simulink model "sim_quadrotor"  (R2015a)
settings: Solver=ode3  StartTime=0  StopTime=inf  FixedStep=sampleTime_qcsim  MaxStep=0.1  RelTol=1e-3
InitFcn:
  | % load parameters of the default quadrotor
  | disp('Quadrotor parameters loaded by InitFcn')
  | paramsFilters %load mdl_quadcopter as well!
  | 
  | % change to Simulation folder if in data folder
  | cd([matlabpath '/Simulation']);
undefined symbols (not defined in the file): altEstim, controlParams, Discrete, ofhandle, quad, quadEDT, sampleTime_qcsim, Time, vishandle
libraries: simulink x25, ctrlSharedLib x3, commnoisgen2 x1
settings Model: CovSFcnEnable=off  Creator=corkep  LastModifiedBy=student
settings DataIOCC: LimitDataPoints=off  SaveFormat=StructureWithTime  SignalLoggingSaveFormat=ModelDataLogs  SignalLogging=off  DSMLogging=off
settings OptimizationCC: ExpressionDepthLimit=2147483647  OptimizeModelRefInitCode=on  LifeSpan=1
settings DebuggingCC: UnderspecifiedInitializationDetection=Classic  MergeDetectMultiDrivingBlocksExec=none  SolverPrmCheckMsg=warning  FcnCallInpInsideContextMsg=UseLocalSettings  StateNameClashWarn=warning
settings HardwareCC: TargetBitPerLong=64  TargetBitPerPointer=64  TargetLongLongMode=on  TargetIntDivRoundTo=Zero  TargetEndianess=LittleEndian  TargetWordSize=64  TargetHWDeviceType=MATLAB Host  ProdEqTarget=off
settings RTWCC: SystemTargetFile=ert_shrlib.tlc  GenCodeOnly=on  MakeCommand="make_rtw OPTS=\"-DDEFAULT_BUFFER_SIZE=4600\""  GenerateMakefile=off  TemplateMakefile=ert_default_tmf  Description=Embedded Coder (host-based shared library target)  BuildConfiguration=Faster Runs  RTWCompilerOptimization=on
settings CodeAppCC: IgnoreCustomStorageClasses=off
settings STFCustomTargetCC: ParMdlRefBuildCompliant=on  CompOptLevelCompliant=on  IncludeMdlTerminateFcn=off  CombineOutputUpdateFcns=on  MatFileLogging=on  MultiInstanceERTCode=on  CodeInterfacePackaging=Reusable function  SupportContinuousTime=off  SupportVariableSizeSignals=off  ModelStepFunctionPrototypeControlCompliant=on  SystemTargetFile=ert_shrlib.tlc
settings ERTTargetCC: ParMdlRefBuildCompliant=on  CompOptLevelCompliant=on  IncludeMdlTerminateFcn=off  MatFileLogging=on  MultiInstanceERTCode=on  CodeInterfacePackaging=Reusable function  SupportContinuousTime=off  SupportVariableSizeSignals=off  ModelStepFunctionPrototypeControlCompliant=on  MultiInstanceErrorCode=Warning  ERTCustomFileTemplate=example_file_process.tlc

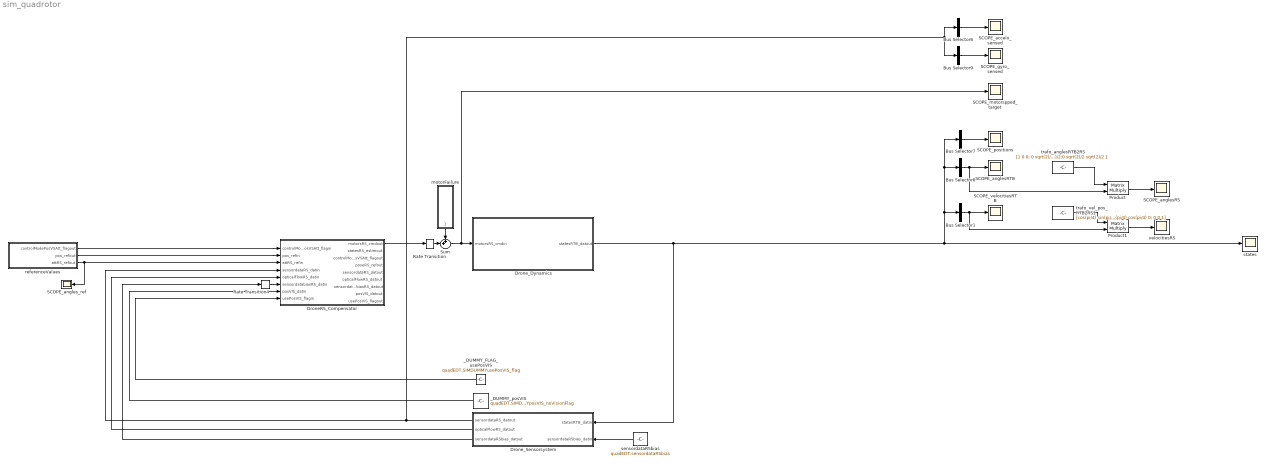
== system sim_quadrotor ==
  Bus Selector1 : BusSelector  OutputSignals=dx,dy,dz  OutputAsBus=on
  Bus Selector6 : BusSelector  OutputSignals=ddx,ddy,ddz  OutputAsBus=on
  Bus Selector7 : BusSelector  OutputSignals=X,Y,Z  OutputAsBus=on
  Bus Selector8 : BusSelector  OutputSignals=yaw,pitch,roll  OutputAsBus=on
  Bus Selector9 : BusSelector  OutputSignals=p,q,r  OutputAsBus=on
  DroneRS_Compensator : Subsystem  TreatAsAtomicUnit=on
  Drone_Dynamics : Subsystem  AncestorBlock=roblocks/Dynamics/Quadrotor
  Drone_Sensorsystem : Subsystem
  Product : Product  Multiplication=Matrix(*)
  Product1 : Product  Multiplication=Matrix(*)
  Rate Transition : RateTransition
  Rate Transition4 : RateTransition  OutPortSampleTime=sampleTime_qcsim
  SCOPE_accelo_sensed : Scope
      settings: TimeRange=14.995  YMin=-13  YMax=2  SaveName=ScopeData11
  SCOPE_anglesRS : Scope
      settings: TimeRange=9.635  YMin=-0.2  YMax=0.1  SaveName=ScopeData8
  SCOPE_anglesRTB : Scope
      settings: TimeRange=10.425  YMin=-0.04  YMax=0.11  SaveName=ScopeData5
  SCOPE_angles_ref : Scope
      settings: TimeRange=15  YMin=-0.15  YMax=0.2  SaveName=ScopeData28
  SCOPE_gyro_sensed : Scope
      settings: TimeRange=14.995  YMin=-0.002  YMax=0.00175  SaveName=ScopeData10
  SCOPE_motorspped_target : Scope
      settings: TimeRange=9.040000000000001  YMin=-400  YMax=400  SaveName=ScopeData2
  SCOPE_positions : Scope
      settings: TimeRange=9.040000000000001  YMin=-1.5  YMax=0.5  SaveName=ScopeData3
  SCOPE_velocitiesRTB : Scope
      settings: TimeRange=13.045  YMin=-1.5  YMax=0.5  SaveName=ScopeData22
  Sum : Sum  Inputs=++|
  _DUMMY_FLAG_usePosVIS : Constant  Value=quadEDT.SIMDUMMYusePosVIS_flag
  _DUMMY_posVIS : Constant  Value=quadEDT.SIMDUMMYposVIS_noVisionFlag
  motorFailure : Subsystem
  referenceValues : Subsystem
  sensordataRSbias : Constant  Value=quadEDT.sensordataRSbias
  states : Scope
      settings: TimeRange=20  YMin=-0.005  YMax=0.055  SaveName=ScopeData7
  trafo_anglesRTB2RS : Constant  Value=[1 0 0; 0 sqrt(2)/2 -sqrt(2)/2;0 sqrt(2)/2 sqrt(2)/2 ]
  trafo_vel_pos_RTB2RS1 : Constant  Value=[cos(pi/4) sin(pi/4) 0 ; -sin(pi/4) cos(pi/4) 0; 0 0 1]
  velocitiesRS : Scope
      settings: TimeRange=8.18  YMin=-4.991831340204151  YMax=1.573556915322435  SaveName=ScopeData39
  wires:
  Bus Selector7/1 -> SCOPE_positions/1
  Bus Selector8/1 -> Product/2, SCOPE_anglesRTB/1
  Bus Selector6/1 -> SCOPE_accelo_sensed/1
  Bus Selector9/1 -> SCOPE_gyro_sensed/1
  DroneRS_Compensator/1(motorsRS_cmdout) -> Rate Transition/1
  referenceValues/2("pos_refout ") -> DroneRS_Compensator/2(pos_refin)
  Sum/1 -> SCOPE_motorspped_target/1, Drone_Dynamics/1(motorsRS_cmdin)
  motorFailure/1(motorRS_cmdout) -> Sum/1
  Rate Transition/1 -> Sum/2
  referenceValues/1(controlModePosVSAtt_flagout) -> DroneRS_Compensator/1(controlModePosVSAtt_flagin)
  referenceValues/3(attRS_refout) -> DroneRS_Compensator/3(attRS_refin), SCOPE_angles_ref/1
  Drone_Dynamics/1(statesRTB_datout) -> Drone_Sensorsystem/1(statesRTB_datin), states/1, Bus Selector1/1, Bus Selector8/1, Bus Selector7/1
  sensordataRSbias/1 -> Drone_Sensorsystem/2(sensordataRSbias_datin)
  Drone_Sensorsystem/2(opticalFlowRS_datout) -> DroneRS_Compensator/5(opticalFlowRS_datin)
  Rate Transition4/1 -> DroneRS_Compensator/6(sensordatabiasRS_datin)
  Drone_Sensorsystem/1(sensordataRS_datout) -> DroneRS_Compensator/4(sensordataRS_datin), Bus Selector9/1, Bus Selector6/1
  Drone_Sensorsystem/3(sensordataRSbias_datout) -> Rate Transition4/1
  Product/1 -> SCOPE_anglesRS/1
  trafo_anglesRTB2RS/1 -> Product/1
  _DUMMY_posVIS/1 -> DroneRS_Compensator/7(posVIS_datin)
  Bus Selector1/1 -> Product1/2, SCOPE_velocitiesRTB/1
  Product1/1 -> velocitiesRS/1
  _DUMMY_FLAG_usePosVIS/1 -> DroneRS_Compensator/8(usePosVIS_flagin)
  trafo_vel_pos_RTB2RS1/1 -> Product1/1

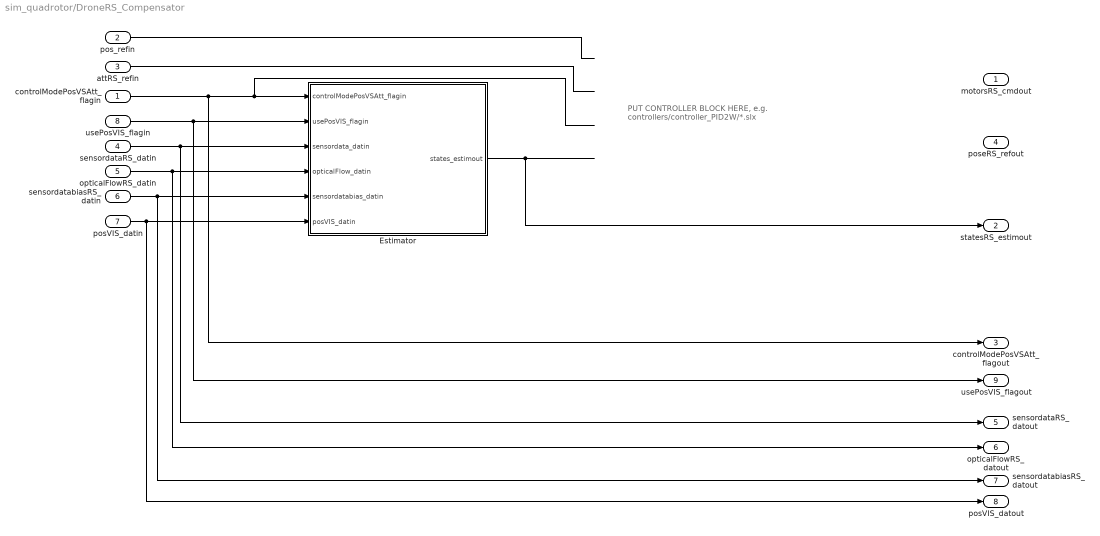
== system sim_quadrotor/DroneRS_Compensator ==
  note: PUT CONTROLLER BLOCK HERE,
      | e.g. controllers/controller_PID2W/*.slx
  controlModePosVSAtt_flagin : Inport
  pos_refin : Inport  Port=2
  attRS_refin : Inport  Port=3
  sensordataRS_datin : Inport  Port=4
  opticalFlowRS_datin : Inport  Port=5
  sensordatabiasRS_datin : Inport  Port=6
  posVIS_datin : Inport  Port=7
  usePosVIS_flagin : Inport  Port=8
  Estimator : Subsystem
  motorsRS_cmdout : Outport
  statesRS_estimout : Outport  Port=2
  controlModePosVSAtt_flagout : Outport  Port=3
  poseRS_refout : Outport  Port=4
  sensordataRS_datout : Outport  Port=5
  opticalFlowRS_datout : Outport  Port=6
  sensordatabiasRS_datout : Outport  Port=7
  posVIS_datout : Outport  Port=8
  usePosVIS_flagout : Outport  Port=9
  wires:
  sensordataRS_datin/1 -> sensordataRS_datout/1, Estimator/3(sensordata_datin)
  pos_refin/1 -> ?
  Estimator/1(states_estimout) -> statesRS_estimout/1
  attRS_refin/1 -> ?
  controlModePosVSAtt_flagin/1 -> controlModePosVSAtt_flagout/1, Estimator/1(controlModePosVSAtt_flagin)
  sensordatabiasRS_datin/1 -> Estimator/5(sensordatabias_datin), sensordatabiasRS_datout/1
  opticalFlowRS_datin/1 -> Estimator/4(opticalFlow_datin), opticalFlowRS_datout/1
  posVIS_datin/1 -> Estimator/6(posVIS_datin), posVIS_datout/1
  ? -> motorsRS_cmdout/1
  usePosVIS_flagin/1 -> usePosVIS_flagout/1, Estimator/2(usePosVIS_flagin)
  ? -> poseRS_refout/1

== system sim_quadrotor/Drone_Dynamics ==
  motorsRS_cmdin : Inport
  Bus Creator : BusCreator  Inputs='X','Y','Z','yaw','pitch','roll','dx','dy','dz','p','q','r'
  Demux : Demux  Outputs=12
  Dynamics (Robotics Toolbox Peter Corke) : S-Function  FunctionName=quadrotor_dynamics  Parameters=quad
  MotorsRSToW : Subsystem
  statesRTB_datout : Outport
  wires:
  Demux/1 -> Bus Creator/1  "X"
  Demux/3 -> Bus Creator/3  "Z"
  Demux/4 -> Bus Creator/4  "yaw"
  Demux/5 -> Bus Creator/5  "pitch"
  motorsRS_cmdin/1 -> MotorsRSToW/1(motorsRS_cmdin)
  Demux/7 -> Bus Creator/7  "dx"
  Demux/9 -> Bus Creator/9  "dz"
  Demux/2 -> Bus Creator/2  "Y"
  Demux/6 -> Bus Creator/6  "roll"
  Demux/8 -> Bus Creator/8  "dy"
  Bus Creator/1 -> statesRTB_datout/1
  Dynamics (Robotics Toolbox Peter Corke)/1 -> Demux/1
  Demux/10 -> Bus Creator/10  "p"
  Demux/11 -> Bus Creator/11  "q"
  Demux/12 -> Bus Creator/12  "r"
  MotorsRSToW/1(omega_cmdout) -> Dynamics (Robotics Toolbox Peter Corke)/1

== system sim_quadrotor/Drone_Sensorsystem ==
  statesRTB_datin : Inport
  sensordataRSbias_datin : Inport  Port=2
  IMU_Pressure : Subsystem
  Rate Transition1 : RateTransition  OutPortSampleTime=sampleTime_qcsim
  Rate Transition2 : RateTransition  OutPortSampleTime=sampleTime_qcsim
  camera : Subsystem
  sensordataRS_datout : Outport
  opticalFlowRS_datout : Outport  Port=2
  sensordataRSbias_datout : Outport  Port=3
  wires:
  statesRTB_datin/1 -> IMU_Pressure/2(statesRTB_datin), camera/1(statesRTB_datin)
  sensordataRSbias_datin/1 -> sensordataRSbias_datout/1, IMU_Pressure/1(sensordataRSbias_datin)
  Rate Transition2/1 -> sensordataRS_datout/1
  Rate Transition1/1 -> opticalFlowRS_datout/1
  IMU_Pressure/1(sensordataRS_datout) -> Rate Transition2/1
  camera/1(opticalFlowRS_datout) -> Rate Transition1/1

== system sim_quadrotor/motorFailure ==
  Constant : Constant  Value=0
  Constant1 : Constant  Value=0
  Mux1 : Mux
  Step : Step  Time=quadEDT.motorFailure_time  SampleTime=0
  Step1 : Step  Time=quadEDT.motorFailure_time + quadEDT.motorFailure_duration  SampleTime=0
  Sum : Sum  Inputs=|+-
  motorFailure_gainm2 : Gain  Gain=quadEDT.motorFailure_gainm2
  motorFailure_gainm3 : Gain  Gain=quadEDT.motorFailure_gainm3
  motorRS_cmdout : Outport
  wires:
  Step/1 -> Sum/1
  Step1/1 -> Sum/2
  Sum/1 -> motorFailure_gainm3/1, motorFailure_gainm2/1
  Constant/1 -> Mux1/1
  motorFailure_gainm2/1 -> Mux1/2
  motorFailure_gainm3/1 -> Mux1/3
  Constant1/1 -> Mux1/4
  Mux1/1 -> motorRS_cmdout/1

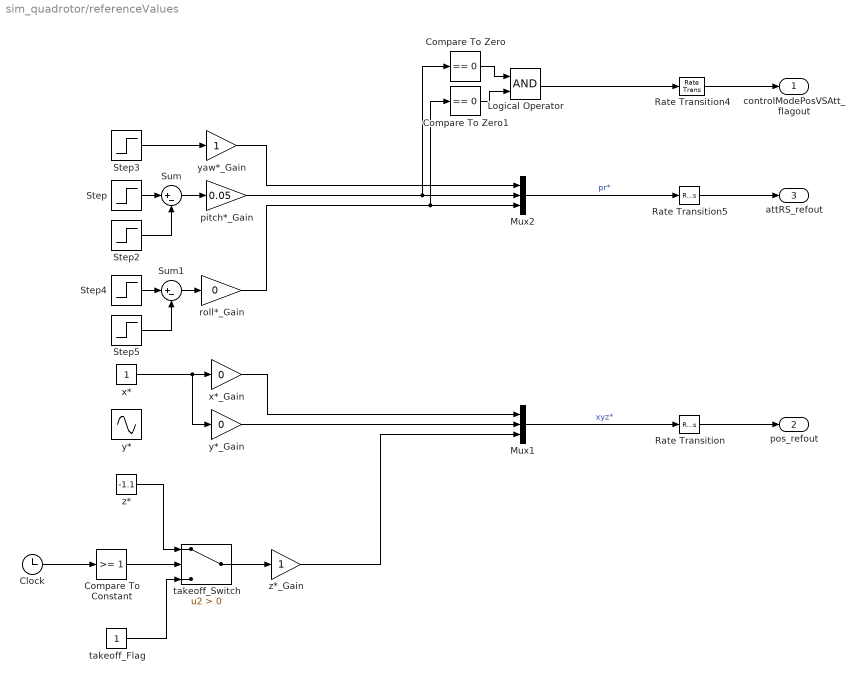
== system sim_quadrotor/referenceValues ==
  Clock : Clock
  Compare To Constant : simulink/Logic and Bit Operations/Compare To Constant  relop=>=  const=1  OutDataTypeStr=boolean
  Compare To Zero : simulink/Logic and Bit Operations/Compare To Zero  relop===  OutDataTypeStr=boolean
  Compare To Zero1 : simulink/Logic and Bit Operations/Compare To Zero  relop===  OutDataTypeStr=boolean
  Logical Operator : Logic  AllPortsSameDT=off  OutDataTypeStr=boolean
  Mux1 : Mux  Inputs=3
  Mux2 : Mux  Inputs=3
  Rate Transition : RateTransition  OutPortSampleTime=sampleTime_qcsim
  Rate Transition4 : RateTransition  OutPortSampleTime=sampleTime_qcsim
  Rate Transition5 : RateTransition  OutPortSampleTime=sampleTime_qcsim
  Step : Step  SampleTime=0
  Step2 : Step  Time=2  SampleTime=0
  Step3 : Step  Time=4.5  After=0.1  SampleTime=0
  Step4 : Step  SampleTime=0
  Step5 : Step  Time=2  SampleTime=0
  Sum : Sum  Inputs=|+-
  Sum1 : Sum  Inputs=|+-
  pitch*_Gain : Gain  Gain=0.05
  roll*_Gain : Gain  Gain=0
  takeoff_Flag : Constant  SampleTime=0
  takeoff_Switch : Switch  Criteria=u2 > Threshold
  x* : Constant  SampleTime=0
  x*_Gain : Gain  Gain=0
  y* : Sin  Frequency=2*pi*.125  SampleTime=0
  y*_Gain : Gain  Gain=0
  yaw*_Gain : Gain
  z* : Constant  Value=-1.1  SampleTime=0
  z*_Gain : Gain
  controlModePosVSAtt_flagout : Outport
  "pos_refout " : Outport  Port=2
  attRS_refout : Outport  Port=3
  wires:
  z*/1 -> takeoff_Switch/1
  y*_Gain/1 -> Mux1/2
  x*/1 -> y*_Gain/1, x*_Gain/1
  Mux1/1 -> Rate Transition/1  "xyz*"
  x*_Gain/1 -> Mux1/1
  Rate Transition/1 -> "pos_refout "/1
  Rate Transition4/1 -> controlModePosVSAtt_flagout/1
  Step/1 -> Sum/1
  Mux2/1 -> Rate Transition5/1  "pr*"
  Sum1/1 -> roll*_Gain/1
  Rate Transition5/1 -> attRS_refout/1
  Sum/1 -> pitch*_Gain/1
  Step2/1 -> Sum/2
  yaw*_Gain/1 -> Mux2/1
  pitch*_Gain/1 -> Mux2/2, Compare To Zero/1
  roll*_Gain/1 -> Mux2/3, Compare To Zero1/1
  Compare To Zero/1 -> Logical Operator/1
  Compare To Zero1/1 -> Logical Operator/2
  Logical Operator/1 -> Rate Transition4/1
  Step3/1 -> yaw*_Gain/1
  Clock/1 -> Compare To Constant/1
  Compare To Constant/1 -> takeoff_Switch/2
  takeoff_Flag/1 -> takeoff_Switch/3
  takeoff_Switch/1 -> z*_Gain/1
  z*_Gain/1 -> Mux1/3
  Step4/1 -> Sum1/1
  Step5/1 -> Sum1/2

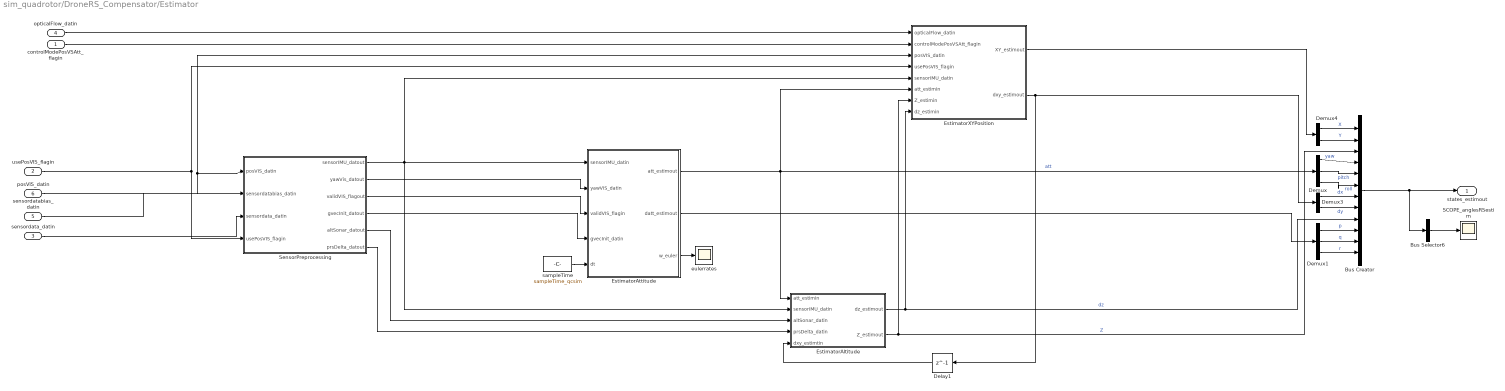
== system sim_quadrotor/DroneRS_Compensator/Estimator ==
  controlModePosVSAtt_flagin : Inport
  usePosVIS_flagin : Inport  Port=2
  sensordata_datin : Inport  Port=3
  opticalFlow_datin : Inport  Port=4
  sensordatabias_datin : Inport  Port=5
  posVIS_datin : Inport  Port=6
  Bus Creator : BusCreator  Inputs='X','Y','Z','yaw','pitch','roll','dx','dy','dz','p','q','r'
  Bus Selector6 : BusSelector  OutputSignals=yaw,pitch,roll  OutputAsBus=on
  Delay1 : Delay  DelayLength=1  InitialCondition=0
  Demux : Demux  Outputs=3
  Demux1 : Demux  Outputs=3
  Demux3 : Demux  Outputs=2
  Demux4 : Demux  Outputs=2
  EstimatorAltitude : Subsystem
  EstimatorAttitude : MATLAB Function  TreatAsAtomicUnit=on
  EstimatorXYPosition : Subsystem
  SCOPE_anglesRSestim : Scope
      settings: TimeRange=3.57  YMin=-0.08  YMax=0.06000000000000001  SaveName=ScopeData4
  SensorPreprocessing : Subsystem
  eulerrates : Scope
      settings: SaveName=ScopeData18
  sampleTime : Constant  Value=sampleTime_qcsim
  states_estimout : Outport
  wires:
  Bus Creator/1 -> Bus Selector6/1, states_estimout/1
  sampleTime/1 -> EstimatorAttitude/5(dt)
  sensordatabias_datin/1 -> SensorPreprocessing/2(sensordatabias_datin)
  EstimatorAttitude/3(w_euler) -> eulerrates/1
  EstimatorAltitude/2(Z_estimout) -> Bus Creator/3, EstimatorXYPosition/7(Z_estimin)  "Z"
  EstimatorAltitude/1(dz_estimout) -> Bus Creator/9, EstimatorXYPosition/8(dz_estimin)  "dz"
  opticalFlow_datin/1 -> EstimatorXYPosition/1(opticalFlow_datin)
  Demux3/1 -> Bus Creator/7  "dx"
  Demux3/2 -> Bus Creator/8  "dy"
  EstimatorXYPosition/2(dxy_estimout) -> Delay1/1, Demux3/1
  Delay1/1 -> EstimatorAltitude/5(dxy_estimtin)
  controlModePosVSAtt_flagin/1 -> EstimatorXYPosition/2(controlModePosVSAtt_flagin)
  Demux4/1 -> Bus Creator/1  "X"
  Demux4/2 -> Bus Creator/2  "Y"
  EstimatorXYPosition/1(XY_estimout) -> Demux4/1
  posVIS_datin/1 -> EstimatorXYPosition/3(posVIS_datin), SensorPreprocessing/1(posVIS_datin)
  usePosVIS_flagin/1 -> SensorPreprocessing/4(usePosVIS_flagin), EstimatorXYPosition/4(usePosVIS_flagin)
  Bus Selector6/1 -> SCOPE_anglesRSestim/1
  SensorPreprocessing/1(sensorIMU_datout) -> EstimatorAltitude/2(sensorIMU_datin), EstimatorXYPosition/5(sensorIMU_datin), EstimatorAttitude/1(sensorIMU_datin)
  SensorPreprocessing/4(gvecInit_datout) -> EstimatorAttitude/4(gvecInit_datin)
  sensordata_datin/1 -> SensorPreprocessing/3(sensordata_datin)
  SensorPreprocessing/5(altSonar_datout) -> EstimatorAltitude/3(altSonar_datin)
  SensorPreprocessing/6(prsDelta_datout) -> EstimatorAltitude/4(prsDelta_datin)
  EstimatorAttitude/1(att_estimout) -> EstimatorAltitude/1(att_estimin), Demux/1, EstimatorXYPosition/6(att_estimin)  "att"
  Demux/1 -> Bus Creator/4  "yaw"
  Demux/2 -> Bus Creator/5  "pitch"
  Demux/3 -> Bus Creator/6  "roll"
  Demux1/1 -> Bus Creator/10  "p"
  Demux1/2 -> Bus Creator/11  "q"
  Demux1/3 -> Bus Creator/12  "r"
  EstimatorAttitude/2(datt_estimout) -> Demux1/1
  SensorPreprocessing/3(validVIS_flagout) -> EstimatorAttitude/3(validVIS_flagin)
  SensorPreprocessing/2(yawVis_datout) -> EstimatorAttitude/2(yawVIS_datin)

== system sim_quadrotor/Drone_Dynamics/MotorsRSToW ==
  motorsRS_cmdin : Inport
  Signed Sqrt : Sqrt  Operator=signedSqrt  SaturateOnIntegerOverflow=on
  motorsRSToW2_Gain : Gain  Gain=quadEDT.motorsRSToW2_Gain
  omega_cmdout : Outport
  wires:
  motorsRSToW2_Gain/1 -> Signed Sqrt/1
  motorsRS_cmdin/1 -> motorsRSToW2_Gain/1
  Signed Sqrt/1 -> omega_cmdout/1

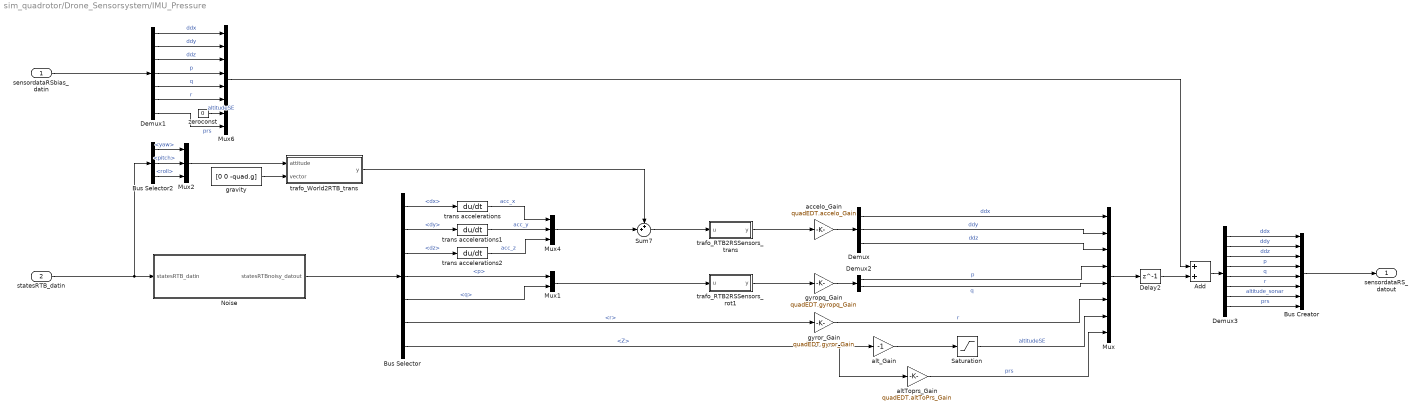
== system sim_quadrotor/Drone_Sensorsystem/IMU_Pressure ==
  sensordataRSbias_datin : Inport
  statesRTB_datin : Inport  Port=2
  " Noise" : Subsystem
  Add : Sum
  Bus Creator : BusCreator  Inputs=8
  Bus Selector : BusSelector  OutputSignals=dx,dy,dz,p,q,r,Z
  Bus Selector2 : BusSelector  OutputSignals=yaw,pitch,roll
  Delay2 : Delay  DelayLength=1  InitialCondition=0
  Demux : Demux  Outputs=3
  Demux1 : Demux  Outputs=7
  Demux2 : Demux  Outputs=2
  Demux3 : Demux  Outputs=8
  Mux : Mux  Inputs=8
  Mux1 : Mux  Inputs=2
  Mux2 : Mux  Inputs=3
  Mux4 : Mux  Inputs=3
  Mux6 : Mux  Inputs=8
  Saturation : Saturate  UpperLimit=inf  LowerLimit=quadEDT.altSenor_LowerLimit
  Sum7 : Sum  Inputs=++|
  accelo_Gain : Gain  Gain=quadEDT.accelo_Gain
  altToprs_Gain : Gain  Gain=quadEDT.altToPrs_Gain
  alt_Gain : Gain  Gain=-1
  gravity : Constant  Value=[0 0 -quad.g]
  gyropq_Gain : Gain  Gain=quadEDT.gyropq_Gain
  gyror_Gain : Gain  Gain=quadEDT.gyror_Gain
  trafo_RTB2RSSensors_rot1 : MATLAB Function  TreatAsAtomicUnit=on
  trafo_RTB2RSSensors_trans : MATLAB Function  TreatAsAtomicUnit=on
  trafo_World2RTB_trans : MATLAB Function  TreatAsAtomicUnit=on
  trans accelerations : Derivative
  trans accelerations1 : Derivative
  trans accelerations2 : Derivative
  zeroconst : Constant  Value=0
  sensordataRS_datout : Outport
  wires:
  statesRTB_datin/1 -> " Noise"/1(statesRTB_datin), Bus Selector2/1
  sensordataRSbias_datin/1 -> Demux1/1
  Demux2/2 -> Mux/5  "q"
  Demux2/1 -> Mux/4  "p"
  " Noise"/1(statesRTBnoisy_datout) -> Bus Selector/1
  Bus Selector/2 -> trans accelerations1/1  "<dy>"
  trans accelerations2/1 -> Mux4/3  "acc_z"
  trafo_RTB2RSSensors_trans/1(y) -> accelo_Gain/1
  Demux/1 -> Mux/1  "ddx"
  Demux/2 -> Mux/2  "ddy"
  gyror_Gain/1 -> Mux/6  "r"
  trans accelerations/1 -> Mux4/1  "acc_x"
  trans accelerations1/1 -> Mux4/2  "acc_y"
  Bus Selector2/1 -> Mux2/1  "<yaw>"
  Bus Selector2/2 -> Mux2/2  "<pitch>"
  Bus Selector2/3 -> Mux2/3  "<roll>"
  Demux/3 -> Mux/3  "ddz"
  Mux2/1 -> trafo_World2RTB_trans/1(attitude)
  gravity/1 -> trafo_World2RTB_trans/2(vector)
  trafo_World2RTB_trans/1(y) -> Sum7/1
  Sum7/1 -> trafo_RTB2RSSensors_trans/1(u)
  Mux4/1 -> Sum7/2
  Mux1/1 -> trafo_RTB2RSSensors_rot1/1(u)
  Bus Selector/4 -> Mux1/1  "<p>"
  Bus Selector/5 -> Mux1/2  "<q>"
  Bus Selector/6 -> gyror_Gain/1  "<r>"
  Bus Selector/7 -> altToprs_Gain/1, alt_Gain/1  "<Z>"
  alt_Gain/1 -> Saturation/1
  Saturation/1 -> Mux/7  "altitudeSE"
  Bus Selector/3 -> trans accelerations2/1  "<dz>"
  altToprs_Gain/1 -> Mux/8  "prs"
  Demux1/1 -> Mux6/1  "ddx"
  Demux1/2 -> Mux6/2  "ddy"
  Demux1/3 -> Mux6/3  "ddz"
  Demux1/4 -> Mux6/4  "p"
  Demux1/5 -> Mux6/5  "q"
  Demux1/6 -> Mux6/6  "r"
  zeroconst/1 -> Mux6/7  "altitudeSE"
  Demux1/7 -> Mux6/8  "prs"
  Mux6/1 -> Add/1
  Add/1 -> Demux3/1
  Mux/1 -> Delay2/1
  Demux3/3 -> Bus Creator/3  "ddz"
  Demux3/1 -> Bus Creator/1  "ddx"
  Demux3/2 -> Bus Creator/2  "ddy"
  Demux3/4 -> Bus Creator/4  "p"
  Demux3/5 -> Bus Creator/5  "q"
  Demux3/6 -> Bus Creator/6  "r"
  Demux3/7 -> Bus Creator/7  "altitude_sonar"
  Demux3/8 -> Bus Creator/8  "prs"
  Bus Creator/1 -> sensordataRS_datout/1
  trafo_RTB2RSSensors_rot1/1(y) -> gyropq_Gain/1
  Bus Selector/1 -> trans accelerations/1  "<dx>"
  Delay2/1 -> Add/2
  accelo_Gain/1 -> Demux/1
  gyropq_Gain/1 -> Demux2/1

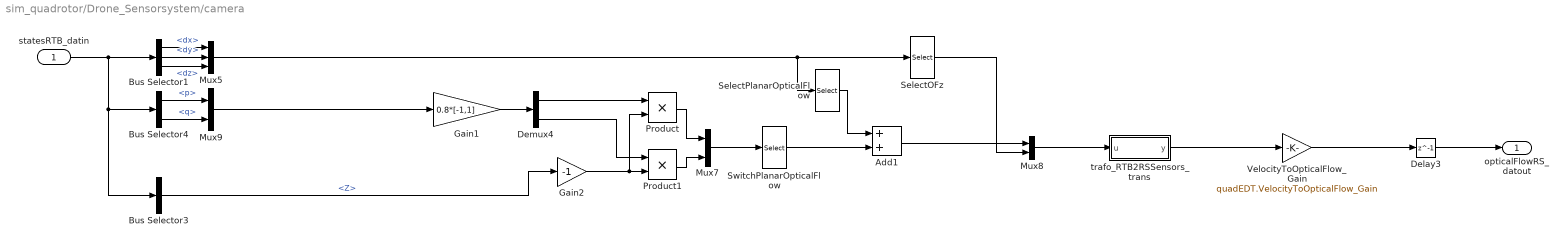
== system sim_quadrotor/Drone_Sensorsystem/camera ==
  statesRTB_datin : Inport
  Add1 : Sum
  Bus Selector1 : BusSelector  OutputSignals=dx,dy,dz
  Bus Selector3 : BusSelector  OutputSignals=Z
  Bus Selector4 : BusSelector  OutputSignals=p,q
  Delay3 : Delay  DelayLength=1  InitialCondition=0
  Demux4 : Demux  Outputs=2
  Gain1 : Gain  Gain=0.8*[-1,1]
  Gain2 : Gain  Gain=-1
  Mux5 : Mux  Inputs=3
  Mux7 : Mux  Inputs=2
  Mux8 : Mux  Inputs=2
  Mux9 : Mux  Inputs=2
  Product : Product
  Product1 : Product
  SelectOFz : Selector  InputPortWidth=3  Indices=3
  SelectPlanarOpticalFlow : Selector  InputPortWidth=3  Indices=[1 2]
  SwitchPlanarOpticalFlow : Selector  InputPortWidth=2  Indices=[2 1]
  VelocityToOpticalFlow_Gain : Gain  Gain=quadEDT.VelocityToOpticalFlow_Gain
  trafo_RTB2RSSensors_trans : MATLAB Function  TreatAsAtomicUnit=on
  opticalFlowRS_datout : Outport
  wires:
  statesRTB_datin/1 -> Bus Selector3/1, Bus Selector4/1, Bus Selector1/1
  Bus Selector1/1 -> Mux5/1  "<dx>"
  Bus Selector1/2 -> Mux5/2  "<dy>"
  Bus Selector1/3 -> Mux5/3  "<dz>"
  VelocityToOpticalFlow_Gain/1 -> Delay3/1
  Mux5/1 -> SelectPlanarOpticalFlow/1, SelectOFz/1
  Demux4/1 -> Product/1
  Gain1/1 -> Demux4/1
  Demux4/2 -> Product1/1
  Product/1 -> Mux7/1
  Product1/1 -> Mux7/2
  Mux7/1 -> SwitchPlanarOpticalFlow/1
  Mux9/1 -> Gain1/1
  Gain2/1 -> Product/2, Product1/2
  SelectPlanarOpticalFlow/1 -> Add1/1
  SwitchPlanarOpticalFlow/1 -> Add1/2
  Add1/1 -> Mux8/1
  SelectOFz/1 -> Mux8/2
  Mux8/1 -> trafo_RTB2RSSensors_trans/1(u)
  Bus Selector3/1 -> Gain2/1  "<Z>"
  Bus Selector4/1 -> Mux9/1  "<p>"
  Bus Selector4/2 -> Mux9/2  "<q>"
  trafo_RTB2RSSensors_trans/1(y) -> VelocityToOpticalFlow_Gain/1
  Delay3/1 -> opticalFlowRS_datout/1

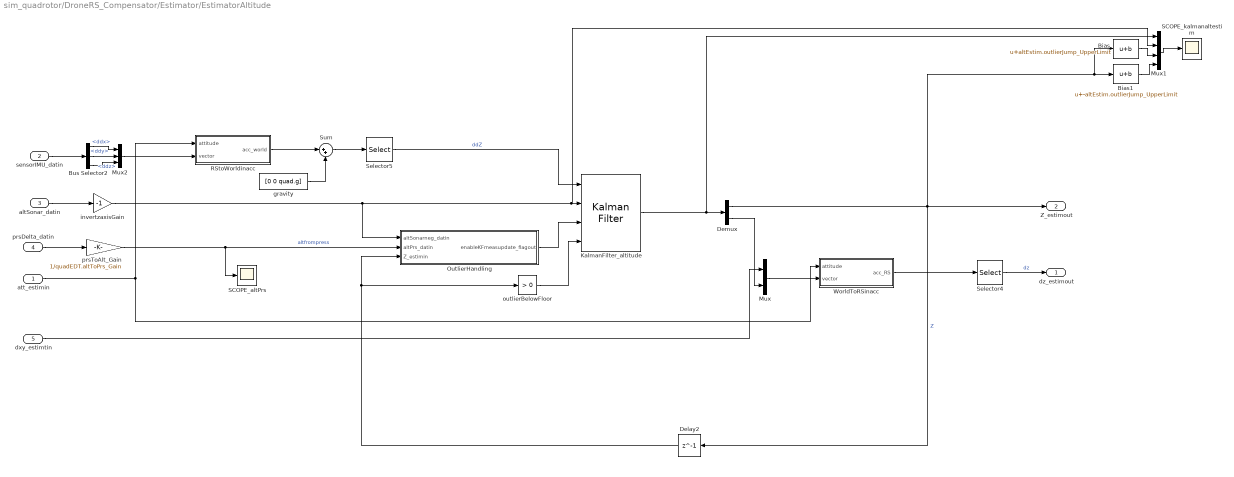
== system sim_quadrotor/DroneRS_Compensator/Estimator/EstimatorAltitude ==
  att_estimin : Inport
  sensorIMU_datin : Inport  Port=2
  altSonar_datin : Inport  Port=3
  prsDelta_datin : Inport  Port=4
  dxy_estimtin : Inport  Port=5
  Bias : Bias  Bias=altEstim.outlierJump_UpperLimit
  Bias1 : Bias  Bias=-altEstim.outlierJump_UpperLimit
  Bus Selector2 : BusSelector  OutputSignals=ddx,ddy,ddz
  Delay2 : Delay  DelayLength=1  InitialCondition=0
  Demux : Demux  Outputs=2
  KalmanFilter_altitude : ctrlSharedLib/Kalman Filter  TimeDomain=Discrete-Time  UseCurrentEstimator=on  ModelSource=Individual A, B, C, D matrices  ModelSourceVariable=sys  A=[1 sampleTime_qcsim; 0 1]  B=[0;sampleTime_qcsim]  C=[1 0]  D=[0]  NumberOfStates=2  NumberOfInputs=2  NumberOfOutputs=2  InitialEstimateSource=Dialog  X0=[-0.046 0]  P0=10  UseK=off  UseGH=on  NumberOfProcessNoiseInputs=2  G=[0;1]  TimeInvariantG=on  H=0  TimeInvariantH=on  Q=0.0005  TimeInvariantQ=on  R=[0.1]  TimeInvariantR=on  N=0  TimeInvariantN=on  AddInputPort=on  AddEnablePort=on  ExternalReset=Level hold  OutputEstimatedY=off  OutputP=off  Ts=-1
  Mux : Mux  Inputs=2
  Mux1 : Mux
  Mux2 : Mux  Inputs=3
  OutlierHandling : Subsystem
  RStoWorldinacc : MATLAB Function  TreatAsAtomicUnit=on
  SCOPE_altPrs : Scope
      settings: TimeRange=10  YMin=-1  YMax=0.4000000000000001  SaveName=ScopeData9
  SCOPE_kalmanaltestim : Scope
      settings: TimeRange=13  YMax=1  SaveName=ScopeData25
  Selector4 : Selector  InputPortWidth=3  Indices=[3]
  Selector5 : Selector  InputPortWidth=3  Indices=[3]
  Sum : Sum  Inputs=|++
  WorldToRSinacc : MATLAB Function  TreatAsAtomicUnit=on
  gravity : Constant  Value=[0 0 quad.g]
  invertzaxisGain : Gain  Gain=-1
  outlierBelowFloor : simulink/Logic and Bit Operations/Compare To Constant  relop=>  const=0  OutDataTypeStr=boolean
  prsToAlt_Gain : Gain  Gain=1/quadEDT.altToPrs_Gain
  dz_estimout : Outport
  Z_estimout : Outport  Port=2
  wires:
  att_estimin/1 -> RStoWorldinacc/1(attitude), WorldToRSinacc/1(attitude)
  altSonar_datin/1 -> invertzaxisGain/1
  RStoWorldinacc/1(acc_world) -> Sum/1
  gravity/1 -> Sum/2
  Sum/1 -> Selector5/1
  KalmanFilter_altitude/1 -> Mux1/1, Demux/1
  Mux/1 -> WorldToRSinacc/2(vector)
  Selector5/1 -> KalmanFilter_altitude/1  "ddZ"
  invertzaxisGain/1 -> Mux1/2, KalmanFilter_altitude/2, OutlierHandling/1(altSonarneg_datin)
  Demux/1 -> Bias1/1, Bias/1, Delay2/1, Z_estimout/1  "Z"
  Selector4/1 -> dz_estimout/1  "dz"
  Demux/2 -> Mux/2
  Mux1/1 -> SCOPE_kalmanaltestim/1
  Bias/1 -> Mux1/3
  Bias1/1 -> Mux1/4
  outlierBelowFloor/1 -> KalmanFilter_altitude/4
  prsDelta_datin/1 -> prsToAlt_Gain/1
  prsToAlt_Gain/1 -> SCOPE_altPrs/1, OutlierHandling/2(altPrs_datin)  "altfrompress"
  Delay2/1 -> outlierBelowFloor/1, OutlierHandling/3(Z_estimin)
  OutlierHandling/1(enableKFmeasupdate_flagout) -> KalmanFilter_altitude/3
  dxy_estimtin/1 -> Mux/1
  WorldToRSinacc/1(acc_RS) -> Selector4/1
  Bus Selector2/1 -> Mux2/1  "<ddx>"
  Bus Selector2/2 -> Mux2/2  "<ddy>"
  Bus Selector2/3 -> Mux2/3  "<ddz>"
  sensorIMU_datin/1 -> Bus Selector2/1
  Mux2/1 -> RStoWorldinacc/2(vector)

== system sim_quadrotor/DroneRS_Compensator/Estimator/EstimatorXYPosition ==
  opticalFlow_datin : Inport
  controlModePosVSAtt_flagin : Inport  Port=2
  posVIS_datin : Inport  Port=3
  usePosVIS_flagin : Inport  Port=4
  sensorIMU_datin : Inport  Port=5
  att_estimin : Inport  Port=6
  Z_estimin : Inport  Port=7
  dz_estimin : Inport  Port=8
  EstimatorVelocity : Subsystem
  EstimatorXYPosition : Subsystem
  XY_estimout : Outport
  dxy_estimout : Outport  Port=2
  wires:
  att_estimin/1 -> EstimatorVelocity/4(att_estimin), EstimatorXYPosition/2(att_estimin)
  EstimatorVelocity/1(dxy_estimout) -> EstimatorXYPosition/1(dxy_estimin), dxy_estimout/1
  opticalFlow_datin/1 -> EstimatorVelocity/1(opticalFlow_datin)
  sensorIMU_datin/1 -> EstimatorVelocity/3(sensorIMU_datin)
  Z_estimin/1 -> EstimatorVelocity/2(Z_estimin)
  controlModePosVSAtt_flagin/1 -> EstimatorXYPosition/3(controlModePosVSAtt_flagin)
  dz_estimin/1 -> EstimatorXYPosition/4(dz_estimin)
  posVIS_datin/1 -> EstimatorXYPosition/5(posVIS_datin)
  usePosVIS_flagin/1 -> EstimatorXYPosition/6(usePosVIS_flagin)
  EstimatorXYPosition/1(XY_estimout) -> XY_estimout/1

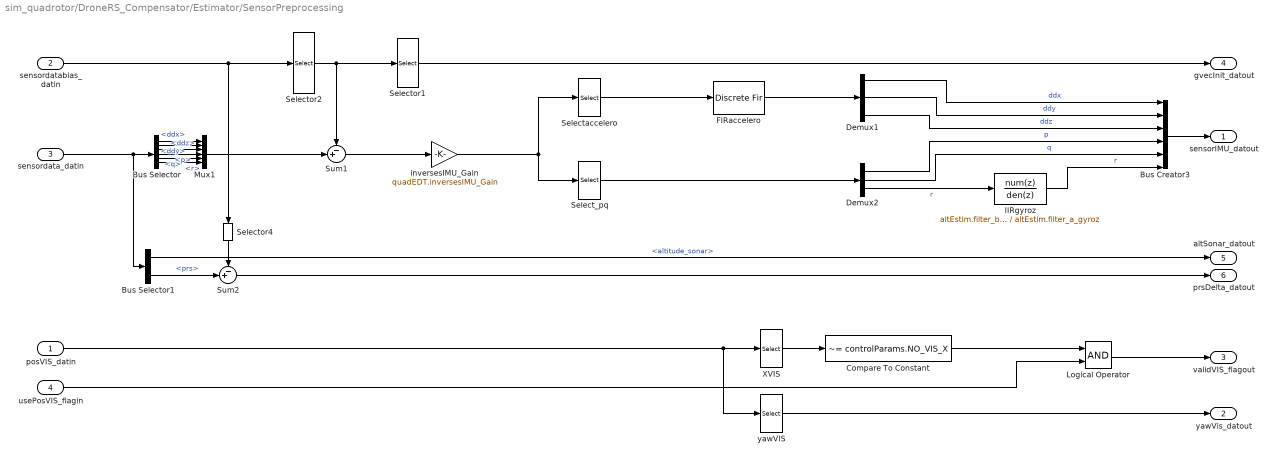
== system sim_quadrotor/DroneRS_Compensator/Estimator/SensorPreprocessing ==
  posVIS_datin : Inport
  sensordatabias_datin : Inport  Port=2
  sensordata_datin : Inport  Port=3
  usePosVIS_flagin : Inport  Port=4
  Bus Creator3 : BusCreator  Inputs=6
  Bus Selector : BusSelector  OutputSignals=ddx,ddy,ddz,p,q,r
  Bus Selector1 : BusSelector  OutputSignals=altitude_sonar,prs
  Compare To Constant : simulink/Logic and Bit Operations/Compare To Constant  relop=~=  const=controlParams.NO_VIS_X  OutDataTypeStr=boolean
  Demux1 : Demux  Outputs=3
  Demux2 : Demux  Outputs=3
  FIRaccelero : DiscreteFir  Coefficients=controlParams.filter_accelero.Coefficients  SampleTime=sampleTime_qcsim
  IIRgyroz : DiscreteFilter  Numerator=altEstim.filter_b_gyroz  Denominator=altEstim.filter_a_gyroz
  Logical Operator : Logic  AllPortsSameDT=off  OutDataTypeStr=boolean
  Mux1 : Mux  Inputs=6
  Select_pq : Selector  InputPortWidth=6  Indices=[4 5 6]
  Selectaccelero : Selector  InputPortWidth=6  Indices=[1 2 3]
  Selector1 : Selector  InputPortWidth=6  Indices=[1:3]
  Selector2 : Selector  InputPortWidth=7  Indices=[1:6]
  Selector4 : Selector  InputPortWidth=7  Indices=[7]
  Sum1 : Sum  Inputs=-+|
  Sum2 : Sum  Inputs=-+|
  XVIS : Selector  InputPortWidth=4
  inversesIMU_Gain : Gain  Gain=quadEDT.inversesIMU_Gain
  yawVIS : Selector  InputPortWidth=4  Indices=4
  sensorIMU_datout : Outport
  yawVis_datout : Outport  Port=2
  validVIS_flagout : Outport  Port=3
  gvecInit_datout : Outport  Port=4
  altSonar_datout : Outport  Port=5
  prsDelta_datout : Outport  Port=6
  wires:
  posVIS_datin/1 -> yawVIS/1, XVIS/1
  Bus Creator3/1 -> sensorIMU_datout/1
  Demux1/1 -> Bus Creator3/1  "ddx"
  Demux1/2 -> Bus Creator3/2  "ddy"
  Demux1/3 -> Bus Creator3/3  "ddz"
  Sum1/1 -> inversesIMU_Gain/1
  Selector2/1 -> Sum1/1, Selector1/1
  Demux2/1 -> Bus Creator3/4  "p"
  Demux2/2 -> Bus Creator3/5  "q"
  inversesIMU_Gain/1 -> Select_pq/1, Selectaccelero/1
  Selectaccelero/1 -> FIRaccelero/1
  FIRaccelero/1 -> Demux1/1
  Demux2/3 -> IIRgyroz/1  "r"
  Selector1/1 -> gvecInit_datout/1
  Select_pq/1 -> Demux2/1
  IIRgyroz/1 -> Bus Creator3/6  "r"
  sensordatabias_datin/1 -> Selector4/1, Selector2/1
  Bus Selector/1 -> Mux1/1  "<ddx>"
  Bus Selector/2 -> Mux1/2  "<ddy>"
  Bus Selector/3 -> Mux1/3  "<ddz>"
  Bus Selector/4 -> Mux1/4  "<p>"
  Bus Selector/5 -> Mux1/5  "<q>"
  Bus Selector/6 -> Mux1/6  "<r>"
  sensordata_datin/1 -> Bus Selector1/1, Bus Selector/1
  Bus Selector1/1 -> altSonar_datout/1  "<altitude_sonar>"
  Selector4/1 -> Sum2/1
  Bus Selector1/2 -> Sum2/2  "<prs>"
  Sum2/1 -> prsDelta_datout/1
  Mux1/1 -> Sum1/2
  XVIS/1 -> Compare To Constant/1
  yawVIS/1 -> yawVis_datout/1
  Logical Operator/1 -> validVIS_flagout/1
  Compare To Constant/1 -> Logical Operator/1
  usePosVIS_flagin/1 -> Logical Operator/2

== system sim_quadrotor/Drone_Sensorsystem/IMU_Pressure/ Noise ==
  statesRTB_datin : Inport
  Add : Sum
  Bus Creator : BusCreator  Inputs='X','Y','Z','yaw','pitch','roll','dx','dy','dz','p','q','r'
  Bus to Vector : BusToVector
  Demux1 : Demux  Outputs=12
  Gaussian Noise Generator : commnoisgen2/Gaussian Noise Generator  m=0  d=quadEDT.noiseStatesSensed_std.^2  s=41  Ts=sampleTime_qcsim  frameBased=off  sampPerFrame=1  orient=off  outDataType=double
  noiseWeights_Gain : Gain  Gain=quadEDT.noiseStatesSensed_weights
  statesRTBnoisy_datout : Outport
  wires:
  Bus Creator/1 -> statesRTBnoisy_datout/1
  Gaussian Noise Generator/1 -> noiseWeights_Gain/1
  Demux1/6 -> Bus Creator/6  "roll"
  Add/1 -> Demux1/1
  Demux1/8 -> Bus Creator/8  "dy"
  Demux1/10 -> Bus Creator/10  "p"
  Demux1/12 -> Bus Creator/12  "r"
  Demux1/2 -> Bus Creator/2  "Y"
  Bus to Vector/1 -> Add/1
  Demux1/3 -> Bus Creator/3  "Z"
  Demux1/7 -> Bus Creator/7  "dx"
  Demux1/9 -> Bus Creator/9  "dz"
  Demux1/4 -> Bus Creator/4  "yaw"
  Demux1/11 -> Bus Creator/11  "q"
  statesRTB_datin/1 -> Bus to Vector/1
  Demux1/5 -> Bus Creator/5  "pitch"
  Demux1/1 -> Bus Creator/1  "X"
  noiseWeights_Gain/1 -> Add/2

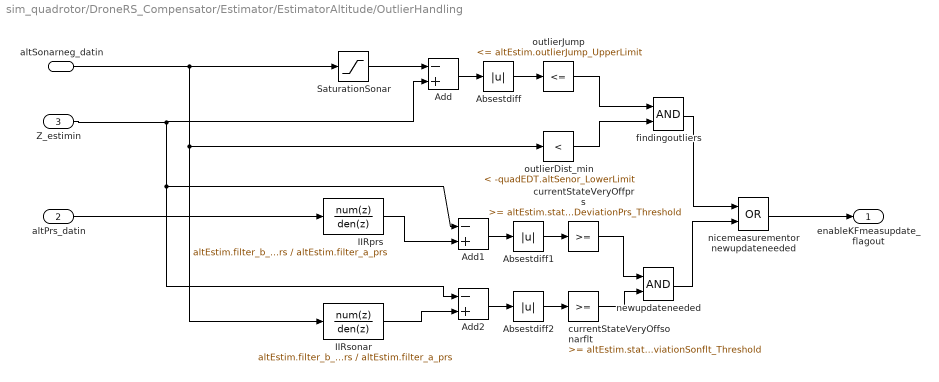
== system sim_quadrotor/DroneRS_Compensator/Estimator/EstimatorAltitude/OutlierHandling ==
  altSonarneg_datin : Inport
  altPrs_datin : Inport  Port=2
  Z_estimin : Inport  Port=3
  Absestdiff : Abs
  Absestdiff1 : Abs
  Absestdiff2 : Abs
  Add : Sum  Inputs=-+
  Add1 : Sum  Inputs=-+
  Add2 : Sum  Inputs=-+
  IIRprs : DiscreteFilter  Numerator=altEstim.filter_b_prs  Denominator=altEstim.filter_a_prs
  IIRsonar : DiscreteFilter  Numerator=altEstim.filter_b_prs  Denominator=altEstim.filter_a_prs
  SaturationSonar : Saturate  UpperLimit=-quadEDT.altSenor_LowerLimit  LowerLimit=-inf
  currentStateVeryOffprs : simulink/Logic and Bit Operations/Compare To Constant  relop=>=  const=altEstim.stateDeviationPrs_Threshold  OutDataTypeStr=boolean
  currentStateVeryOffsonarflt : simulink/Logic and Bit Operations/Compare To Constant  relop=>=  const=altEstim.stateDeviationSonflt_Threshold  OutDataTypeStr=boolean
  findingoutliers : Logic  AllPortsSameDT=off  OutDataTypeStr=boolean
  newupdateneeded : Logic  AllPortsSameDT=off  OutDataTypeStr=boolean
  nicemeasurementor newupdateneeded : Logic  Operator=OR  AllPortsSameDT=off  OutDataTypeStr=boolean
  outlierDist_min : simulink/Logic and Bit Operations/Compare To Constant  relop=<  const=-quadEDT.altSenor_LowerLimit  OutDataTypeStr=boolean
  outlierJump : simulink/Logic and Bit Operations/Compare To Constant  relop=<=  const=altEstim.outlierJump_UpperLimit  OutDataTypeStr=boolean
  enableKFmeasupdate_flagout : Outport
  wires:
  Absestdiff1/1 -> currentStateVeryOffprs/1
  IIRsonar/1 -> Add2/2
  altPrs_datin/1 -> IIRprs/1
  IIRprs/1 -> Add1/2
  currentStateVeryOffsonarflt/1 -> newupdateneeded/2
  Add2/1 -> Absestdiff2/1
  Z_estimin/1 -> Add2/1, Add1/1, Add/2
  currentStateVeryOffprs/1 -> newupdateneeded/1
  altSonarneg_datin/1 -> outlierDist_min/1, IIRsonar/1, SaturationSonar/1
  Absestdiff2/1 -> currentStateVeryOffsonarflt/1
  newupdateneeded/1 -> nicemeasurementor newupdateneeded/2
  Add/1 -> Absestdiff/1
  Absestdiff/1 -> outlierJump/1
  SaturationSonar/1 -> Add/1
  outlierJump/1 -> findingoutliers/1
  outlierDist_min/1 -> findingoutliers/2
  findingoutliers/1 -> nicemeasurementor newupdateneeded/1
  nicemeasurementor newupdateneeded/1 -> enableKFmeasupdate_flagout/1
  Add1/1 -> Absestdiff1/1

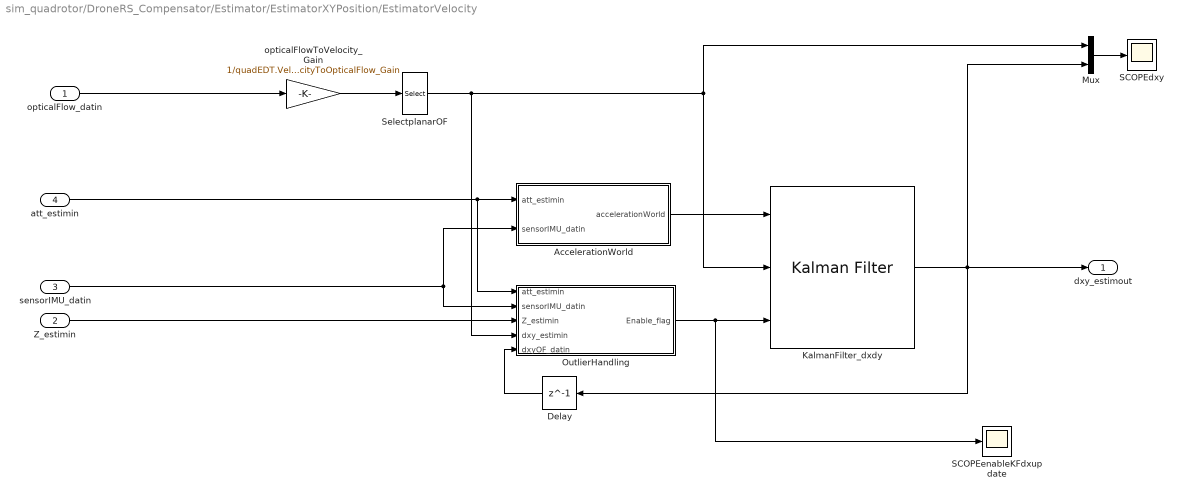
== system sim_quadrotor/DroneRS_Compensator/Estimator/EstimatorXYPosition/EstimatorVelocity ==
  opticalFlow_datin : Inport
  Z_estimin : Inport  Port=2
  sensorIMU_datin : Inport  Port=3
  att_estimin : Inport  Port=4
  AccelerationWorld : Subsystem
  Delay : Delay  DelayLength=1  InitialCondition=0
  KalmanFilter_dxdy : ctrlSharedLib/Kalman Filter  TimeDomain=Discrete-Time  UseCurrentEstimator=on  ModelSource=Individual A, B, C, D matrices  ModelSourceVariable=ss(0.95,1,1,0,1)  A=eye(2)  B=sampleTime_qcsim*eye(2)  C=eye(2)  D=0  NumberOfStates=1  NumberOfInputs=1  NumberOfOutputs=1  InitialEstimateSource=Dialog  X0=0  P0=10  UseK=off  UseGH=on  NumberOfProcessNoiseInputs=1  G=eye(2)  TimeInvariantG=on  H=0  TimeInvariantH=on  Q=0.09.*eye(2)  TimeInvariantQ=on  R=5*eye(2)  TimeInvariantR=on  N=0  TimeInvariantN=on  AddInputPort=on  AddEnablePort=on  OutputEstimatedY=off  OutputP=off  Ts=-1
  Mux : Mux  Inputs=2
  OutlierHandling : Subsystem
  SCOPEdxy : Scope
      settings: TimeRange=2.5  YMin=-12  YMax=6
  SCOPEenableKFdxupdate : Scope
      settings: TimeRange=2.2  YMin=0  YMax=1
  SelectplanarOF : Selector  InputPortWidth=3  Indices=[1 2]
  opticalFlowToVelocity_Gain : Gain  Gain=1/quadEDT.VelocityToOpticalFlow_Gain
  dxy_estimout : Outport
  wires:
  att_estimin/1 -> OutlierHandling/1(att_estimin), AccelerationWorld/1(att_estimin)
  sensorIMU_datin/1 -> AccelerationWorld/2(sensorIMU_datin), OutlierHandling/2(sensorIMU_datin)
  opticalFlow_datin/1 -> opticalFlowToVelocity_Gain/1
  SelectplanarOF/1 -> OutlierHandling/4(dxy_estimin), KalmanFilter_dxdy/2, Mux/1
  opticalFlowToVelocity_Gain/1 -> SelectplanarOF/1
  KalmanFilter_dxdy/1 -> Mux/2, dxy_estimout/1, Delay/1
  OutlierHandling/1(Enable_flag) -> SCOPEenableKFdxupdate/1, KalmanFilter_dxdy/3
  Z_estimin/1 -> OutlierHandling/3(Z_estimin)
  Mux/1 -> SCOPEdxy/1
  AccelerationWorld/1(accelerationWorld) -> KalmanFilter_dxdy/1
  Delay/1 -> OutlierHandling/5(dxyOF_datin)

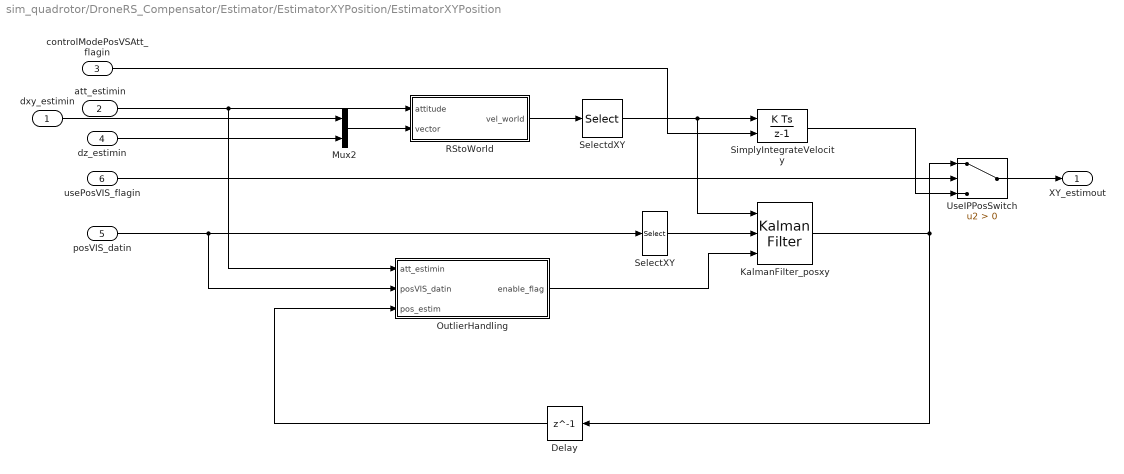
== system sim_quadrotor/DroneRS_Compensator/Estimator/EstimatorXYPosition/EstimatorXYPosition ==
  dxy_estimin : Inport
  att_estimin : Inport  Port=2
  controlModePosVSAtt_flagin : Inport  Port=3
  dz_estimin : Inport  Port=4
  posVIS_datin : Inport  Port=5
  usePosVIS_flagin : Inport  Port=6
  Delay : Delay  DelayLength=1  InitialCondition=0
  KalmanFilter_posxy : ctrlSharedLib/Kalman Filter  TimeDomain=Discrete-Time  UseCurrentEstimator=on  ModelSource=Individual A, B, C, D matrices  ModelSourceVariable=ss(0.95,1,1,0,1)  A=eye(2)  B=sampleTime_qcsim*eye(2)  C=eye(2)  D=0  NumberOfStates=1  NumberOfInputs=1  NumberOfOutputs=1  InitialEstimateSource=Dialog  X0=[.1 0.0]  P0=10  UseK=off  UseGH=on  NumberOfProcessNoiseInputs=1  G=0.1*eye(2)  TimeInvariantG=on  H=0  TimeInvariantH=on  Q=0.001*eye(2)  TimeInvariantQ=on  R=0.3*eye(2)  TimeInvariantR=on  N=0  TimeInvariantN=on  AddInputPort=on  AddEnablePort=on  OutputEstimatedY=off  OutputP=off  Ts=-1
  Mux2 : Mux  Inputs=2
  OutlierHandling : Subsystem
  RStoWorld : MATLAB Function  TreatAsAtomicUnit=on
  SelectXY : Selector  InputPortWidth=4  Indices=[1 2]
  SelectdXY : Selector  InputPortWidth=3  Indices=[1 2]
  SimplyIntegrateVelocity : DiscreteIntegrator  ExternalReset=rising  InitialConditionSetting=State (most efficient)  SampleTime=sampleTime_qcsim  LimitOutput=on  UpperSaturationLimit=2  LowerSaturationLimit=-2
  UseIPPosSwitch : Switch  Criteria=u2 > Threshold
  XY_estimout : Outport
  wires:
  att_estimin/1 -> RStoWorld/1(attitude), OutlierHandling/1(att_estimin)
  dxy_estimin/1 -> Mux2/1
  SimplyIntegrateVelocity/1 -> UseIPPosSwitch/3
  dz_estimin/1 -> Mux2/2
  Mux2/1 -> RStoWorld/2(vector)
  RStoWorld/1(vel_world) -> SelectdXY/1
  SelectdXY/1 -> KalmanFilter_posxy/1, SimplyIntegrateVelocity/1
  posVIS_datin/1 -> SelectXY/1, OutlierHandling/2(posVIS_datin)
  KalmanFilter_posxy/1 -> Delay/1, UseIPPosSwitch/1
  controlModePosVSAtt_flagin/1 -> SimplyIntegrateVelocity/2
  UseIPPosSwitch/1 -> XY_estimout/1
  usePosVIS_flagin/1 -> UseIPPosSwitch/2
  SelectXY/1 -> KalmanFilter_posxy/2
  OutlierHandling/1(enable_flag) -> KalmanFilter_posxy/3
  Delay/1 -> OutlierHandling/3(pos_estim)

== system sim_quadrotor/DroneRS_Compensator/Estimator/EstimatorXYPosition/EstimatorVelocity/AccelerationWorld ==
  note: selectaccelero
  att_estimin : Inport
  sensorIMU_datin : Inport  Port=2
  Add : Sum  Inputs=-+
  Bus Selector1 : BusSelector  OutputSignals=ddx,ddy,ddz
  Mux6 : Mux  Inputs=3
  SelectPlanarddxy : Selector  InputPortWidth=3  Indices=[1 2]
  World2Body : MATLAB Function  TreatAsAtomicUnit=on
  gainaccinput : Gain  Gain=0.2
  gravity : Constant  Value=[0 0 -quad.g]
  accelerationWorld : Outport
  wires:
  att_estimin/1 -> World2Body/1(attitude)
  Bus Selector1/2 -> Mux6/2  "<ddy>"
  Mux6/1 -> Add/2
  sensorIMU_datin/1 -> Bus Selector1/1
  Bus Selector1/1 -> Mux6/1  "<ddx>"
  Bus Selector1/3 -> Mux6/3  "<ddz>"
  SelectPlanarddxy/1 -> gainaccinput/1
  gainaccinput/1 -> accelerationWorld/1
  gravity/1 -> World2Body/2(vector)
  World2Body/1(y) -> Add/1
  Add/1 -> SelectPlanarddxy/1

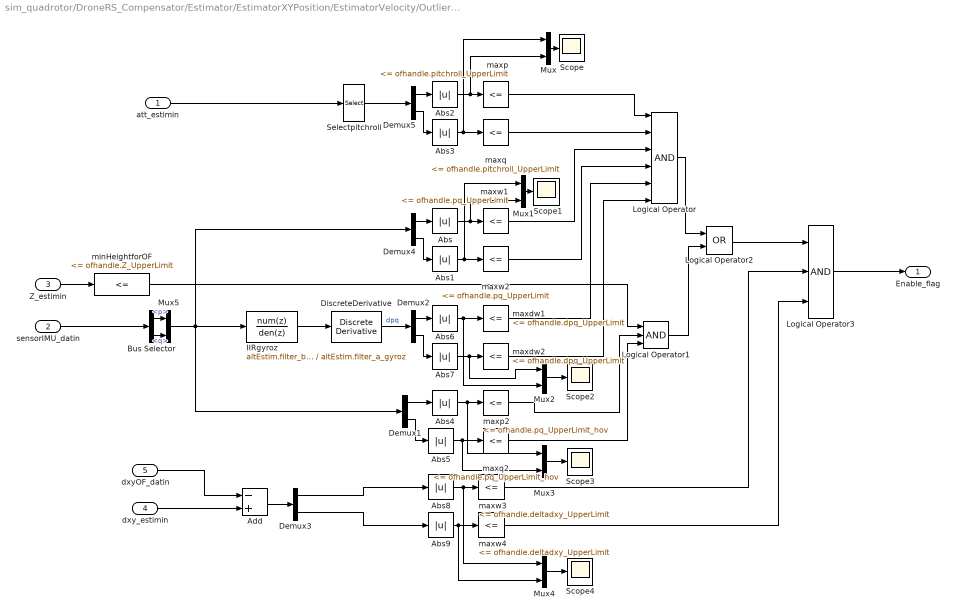
== system sim_quadrotor/DroneRS_Compensator/Estimator/EstimatorXYPosition/EstimatorVelocity/OutlierHandling ==
  att_estimin : Inport
  sensorIMU_datin : Inport  Port=2
  Z_estimin : Inport  Port=3
  dxy_estimin : Inport  Port=4
  dxyOF_datin : Inport  Port=5
  Abs{,1..9} (10 alike) : Abs
  Add : Sum  Inputs=-+
  Bus Selector : BusSelector  OutputSignals=p,q
  Demux{1..5} (5 alike) : Demux  Outputs=2
  DiscreteDerivative : simulink/Discrete/Discrete Derivative  gainval=1.0  ICPrevScaledInput=0.0  InputProcessing=Inherited  OutMin=[]  OutMax=[]  OutDataType=fixdt(1, 16)  OutScaling=2^-10  DoSatur=off
  IIRgyroz : DiscreteFilter  Numerator=altEstim.filter_b_gyroz  Denominator=altEstim.filter_a_gyroz
  Logical Operator : Logic  Inputs=6  AllPortsSameDT=off  OutDataTypeStr=boolean
  Logical Operator1 : Logic  Inputs=3  AllPortsSameDT=off  OutDataTypeStr=boolean
  Logical Operator2 : Logic  Operator=OR  AllPortsSameDT=off  OutDataTypeStr=boolean
  Logical Operator3 : Logic  Inputs=3  AllPortsSameDT=off  OutDataTypeStr=boolean
  Mux{,1..5} (6 alike) : Mux  Inputs=2
  Scope{,1..4} (5 alike) : Scope
      Scope settings: SaveName=ScopeData2
      Scope1 settings: SaveName=ScopeData3
      Scope2 settings: SaveName=ScopeData5
      Scope3 settings: SaveName=ScopeData6
      Scope4 settings: SaveName=ScopeData7
  Selectpitchroll : Selector  InputPortWidth=3  Indices=[2 3]
  maxdw1 : simulink/Logic and Bit Operations/Compare To Constant  relop=<=  const=ofhandle.dpq_UpperLimit  OutDataTypeStr=boolean
  maxdw2 : simulink/Logic and Bit Operations/Compare To Constant  relop=<=  const=ofhandle.dpq_UpperLimit  OutDataTypeStr=boolean
  maxp : simulink/Logic and Bit Operations/Compare To Constant  relop=<=  const=ofhandle.pitchroll_UpperLimit  OutDataTypeStr=boolean
  maxp2 : simulink/Logic and Bit Operations/Compare To Constant  relop=<=  const=ofhandle.pq_UpperLimit_hov  OutDataTypeStr=boolean
  maxq : simulink/Logic and Bit Operations/Compare To Constant  relop=<=  const=ofhandle.pitchroll_UpperLimit  OutDataTypeStr=boolean
  maxq2 : simulink/Logic and Bit Operations/Compare To Constant  relop=<=  const=ofhandle.pq_UpperLimit_hov  OutDataTypeStr=boolean
  maxw1 : simulink/Logic and Bit Operations/Compare To Constant  relop=<=  const=ofhandle.pq_UpperLimit  OutDataTypeStr=boolean
  maxw2 : simulink/Logic and Bit Operations/Compare To Constant  relop=<=  const=ofhandle.pq_UpperLimit  OutDataTypeStr=boolean
  maxw3 : simulink/Logic and Bit Operations/Compare To Constant  relop=<=  const=ofhandle.deltadxy_UpperLimit  OutDataTypeStr=boolean
  maxw4 : simulink/Logic and Bit Operations/Compare To Constant  relop=<=  const=ofhandle.deltadxy_UpperLimit  OutDataTypeStr=boolean
  minHeightforOF : simulink/Logic and Bit Operations/Compare To Constant  relop=<=  const=ofhandle.Z_UpperLimit  OutDataTypeStr=boolean
  Enable_flag : Outport
  wires:
  maxp2/1 -> Logical Operator1/2
  Demux5/2 -> Abs3/1
  minHeightforOF/1 -> Logical Operator1/1
  Demux5/1 -> Abs2/1
  maxq/1 -> Logical Operator/2
  maxdw2/1 -> Logical Operator/6
  maxdw1/1 -> Logical Operator/5
  att_estimin/1 -> Selectpitchroll/1
  maxw2/1 -> Logical Operator/4
  maxp/1 -> Logical Operator/1
  Bus Selector/2 -> Mux5/2  "<q>"
  maxq2/1 -> Logical Operator1/3
  sensorIMU_datin/1 -> Bus Selector/1
  Selectpitchroll/1 -> Demux5/1
  Bus Selector/1 -> Mux5/1  "<p>"
  maxw1/1 -> Logical Operator/3
  Logical Operator/1 -> Logical Operator2/1
  Z_estimin/1 -> minHeightforOF/1
  Abs/1 -> Mux1/2, maxw1/1
  Abs1/1 -> Mux1/1, maxw2/1
  Demux4/1 -> Abs/1
  Demux4/2 -> Abs1/1
  Abs2/1 -> Mux/2, maxp/1
  Abs3/1 -> Mux/1, maxq/1
  Abs4/1 -> Mux3/1, maxp2/1
  Abs5/1 -> Mux3/2, maxq2/1
  Demux1/1 -> Abs4/1
  Demux1/2 -> Abs5/1
  Logical Operator1/1 -> Logical Operator2/2
  Abs6/1 -> Mux2/2, maxdw1/1
  Abs7/1 -> Mux2/1, maxdw2/1
  Demux2/1 -> Abs6/1
  Demux2/2 -> Abs7/1
  DiscreteDerivative/1 -> Demux2/1  "dpq"
  Logical Operator3/1 -> Enable_flag/1
  Logical Operator2/1 -> Logical Operator3/1
  Abs8/1 -> Mux4/1, maxw3/1
  Abs9/1 -> Mux4/2, maxw4/1
  Add/1 -> Demux3/1
  dxy_estimin/1 -> Add/2
  Demux3/1 -> Abs8/1
  Demux3/2 -> Abs9/1
  dxyOF_datin/1 -> Add/1
  maxw3/1 -> Logical Operator3/2
  maxw4/1 -> Logical Operator3/3
  Mux/1 -> Scope/1
  Mux1/1 -> Scope1/1
  Mux2/1 -> Scope2/1
  Mux3/1 -> Scope3/1
  Mux4/1 -> Scope4/1
  Mux5/1 -> Demux4/1, Demux1/1, IIRgyroz/1
  IIRgyroz/1 -> DiscreteDerivative/1

== system sim_quadrotor/DroneRS_Compensator/Estimator/EstimatorXYPosition/EstimatorXYPosition/OutlierHandling ==
  att_estimin : Inport
  posVIS_datin : Inport  Port=2
  pos_estim : Inport  Port=3
  Add1 : Sum  Inputs=+-
  Demux6 : Demux  Outputs=3
  Logical Operator3 : Logic  Inputs=4  AllPortsSameDT=off  OutDataTypeStr=boolean
  SelectX : Selector  InputPortWidth=4  Indices=[1]
  SelectXY : Selector  InputPortWidth=4  Indices=[1 2]
  abs : MATLAB Function  TreatAsAtomicUnit=on
  checkPosavailable : simulink/Logic and Bit Operations/Compare To Constant  relop=~=  const=-99  OutDataTypeStr=boolean
  maxp3 : simulink/Logic and Bit Operations/Compare To Constant  relop=<=  const=vishandle.att_UpperLimit  OutDataTypeStr=boolean
  maxq3 : simulink/Logic and Bit Operations/Compare To Constant  relop=<=  const=vishandle.att_UpperLimit  OutDataTypeStr=boolean
  planarjumpsVISPOS : simulink/Logic and Bit Operations/Compare To Constant  relop=<  const=vishandle.deltaXY  OutDataTypeStr=boolean
  enable_flag : Outport
  wires:
  att_estimin/1 -> Demux6/1
  posVIS_datin/1 -> SelectXY/1, SelectX/1
  SelectX/1 -> checkPosavailable/1
  checkPosavailable/1 -> Logical Operator3/1
  Logical Operator3/1 -> enable_flag/1
  Demux6/2 -> maxp3/1
  Demux6/3 -> maxq3/1
  maxp3/1 -> Logical Operator3/2
  maxq3/1 -> Logical Operator3/3
  SelectXY/1 -> Add1/1
  Add1/1 -> abs/1(vec)
  pos_estim/1 -> Add1/2
  abs/1(y) -> planarjumpsVISPOS/1
  planarjumpsVISPOS/1 -> Logical Operator3/4

== matlab function sim_quadrotor/Drone_Sensorsystem/camera/trafo_RTB2RSSensors_trans ==
  data: u input; y output
function y = fcn(u)
%inverse yaw-rotation
y = ([cos(pi/4) sin(pi/4) 0 ; -sin(pi/4) cos(pi/4) 0; 0 0 1]*u);

== matlab function sim_quadrotor/Drone_Sensorsystem/IMU_Pressure/trafo_RTB2RSSensors_trans ==
  data: u input; y output
function y = fcn(u)
%inverse yaw-rotation
y = ([cos(pi/4) sin(pi/4) 0 ; -sin(pi/4) cos(pi/4) 0; 0 0 1]*u);

== matlab function sim_quadrotor/Drone_Sensorsystem/IMU_Pressure/trafo_RTB2RSSensors_rot1 ==
  data: u input; y output
function y = fcn(u)
%inverse yaw-rotation
y = [cos(pi/4)  sin(pi/4); -sin(pi/4) cos(pi/4)]*u;

== matlab function sim_quadrotor/DroneRS_Compensator/Estimator/EstimatorXYPosition/EstimatorVelocity/AccelerationWorld/World2Body ==
  data: attitude input; vector input; y output
function y = fcn(attitude,vector)

yaw = attitude(1);
pitch = attitude(2);
roll = attitude(3);

% rotz(yaw)*roty(pitch)*rotx(roll)
%     R_RTBBodytoGlobal = [cos(pitch)*cos(yaw) sin(roll)*sin(pitch)*cos(yaw)-cos(roll)*sin(yaw) cos(roll)*sin(pitch)*cos(yaw)+sin(roll)*sin(yaw);   %BBF > Inertial rotation matrix
%          cos(pitch)*sin(yaw) sin(roll)*sin(pitch)*sin(yaw)+cos(roll)*cos(yaw) cos(roll)*sin(pitch)*sin(yaw)-sin(roll)*cos(yaw);
%          -sin(pitch)         sin(roll)*cos(pitch)                            cos(roll)*cos(pitch)];
    

R_Global2RTBBody = [cos(yaw)*cos(pitch), cos(pitch)*sin(yaw),  -sin(pitch);
    cos(yaw)*sin(roll)*sin(pitch)-cos(roll)*sin(yaw), cos(yaw)*cos(roll)+sin(yaw)*sin(pitch), cos(pitch)*sin(roll);
    sin(yaw)*sin(roll)+cos(yaw)*cos(roll)*sin(pitch), cos(roll)*sin(yaw)*sin(pitch)-cos(yaw)*sin(roll), cos(roll)*cos(pitch)];

% Rw_Global2RTBBody  = [0        sin(roll)          cos(roll);             %inverted Wronskian
%           0        cos(roll)*cos(pitch) -sin(roll)*cos(pitch);
%           cos(pitch) sin(roll)*sin(pitch) cos(roll)*sin(pitch)] / cos(pitch);
      
      
      
 y = R_Global2RTBBody*vector;      
      
%y = -([cos(pi/4) sin(pi/4); -sin(pi/4) cos(pi/4)]*u);

== matlab function sim_quadrotor/Drone_Sensorsystem/IMU_Pressure/trafo_World2RTB_trans ==
  data: attitude input; vector input; y output
function y = fcn(attitude,vector)

yaw = attitude(1);
pitch = attitude(2);
roll = attitude(3);

% rotz(yaw)*roty(pitch)*rotx(roll)
%     R_RTBBodytoGlobal = [cos(pitch)*cos(yaw) sin(roll)*sin(pitch)*cos(yaw)-cos(roll)*sin(yaw) cos(roll)*sin(pitch)*cos(yaw)+sin(roll)*sin(yaw);   %BBF > Inertial rotation matrix
%          cos(pitch)*sin(yaw) sin(roll)*sin(pitch)*sin(yaw)+cos(roll)*cos(yaw) cos(roll)*sin(pitch)*sin(yaw)-sin(roll)*cos(yaw);
%          -sin(pitch)         sin(roll)*cos(pitch)                            cos(roll)*cos(pitch)];
    

R_Global2RTBBody = [cos(yaw)*cos(pitch), cos(pitch)*sin(yaw),  -sin(pitch);
    cos(yaw)*sin(roll)*sin(pitch)-cos(roll)*sin(yaw), cos(yaw)*cos(roll)+sin(yaw)*sin(pitch), cos(pitch)*sin(roll);
    sin(yaw)*sin(roll)+cos(yaw)*cos(roll)*sin(pitch), cos(roll)*sin(yaw)*sin(pitch)-cos(yaw)*sin(roll), cos(roll)*cos(pitch)];

% Rw_Global2RTBBody  = [0        sin(roll)          cos(roll);             %inverted Wronskian
%           0        cos(roll)*cos(pitch) -sin(roll)*cos(pitch);
%           cos(pitch) sin(roll)*sin(pitch) cos(roll)*sin(pitch)] / cos(pitch);
      
      
      
 y = R_Global2RTBBody*vector;      
      
%y = -([cos(pi/4) sin(pi/4); -sin(pi/4) cos(pi/4)]*u);

== matlab function sim_quadrotor/DroneRS_Compensator/Estimator/EstimatorXYPosition/EstimatorXYPosition/RStoWorld ==
  data: attitude input; vector input; vel_world output
function vel_world = fcn(attitude,vector)
yaw = attitude(1);
pitch = attitude(2);
roll = attitude(3);








R_RTBBodytoGlobal = [cos(pitch)*cos(yaw) sin(roll)*sin(pitch)*cos(yaw)-cos(roll)*sin(yaw) cos(roll)*sin(pitch)*cos(yaw)+sin(roll)*sin(yaw);   %BBF > Inertial rotation matrix
  cos(pitch)*sin(yaw) sin(roll)*sin(pitch)*sin(yaw)+cos(roll)*cos(yaw) cos(roll)*sin(pitch)*sin(yaw)-sin(roll)*cos(yaw);
  -sin(pitch)         sin(roll)*cos(pitch)                            cos(roll)*cos(pitch)];

vel_world = R_RTBBodytoGlobal*vector;

== matlab function sim_quadrotor/DroneRS_Compensator/Estimator/EstimatorAltitude/RStoWorldinacc ==
  data: attitude input; vector input; acc_world output
function acc_world = fcn(attitude,vector)
yaw = attitude(1);
pitch = attitude(2);
roll = attitude(3);








R_RTBBodytoGlobal = [cos(pitch)*cos(yaw) sin(roll)*sin(pitch)*cos(yaw)-cos(roll)*sin(yaw) cos(roll)*sin(pitch)*cos(yaw)+sin(roll)*sin(yaw);   %BBF > Inertial rotation matrix
  cos(pitch)*sin(yaw) sin(roll)*sin(pitch)*sin(yaw)+cos(roll)*cos(yaw) cos(roll)*sin(pitch)*sin(yaw)-sin(roll)*cos(yaw);
  -sin(pitch)         sin(roll)*cos(pitch)                            cos(roll)*cos(pitch)];

acc_world = R_RTBBodytoGlobal*vector;

== matlab function sim_quadrotor/DroneRS_Compensator/Estimator/EstimatorAltitude/WorldToRSinacc ==
  data: attitude input; vector input; acc_RS output
function acc_RS = fcn(attitude,vector)
yaw = attitude(1);
pitch = attitude(2);
roll = attitude(3);


R_Global2RTBBody = [cos(yaw)*cos(pitch), cos(pitch)*sin(yaw),  -sin(pitch);
    cos(yaw)*sin(roll)*sin(pitch)-cos(roll)*sin(yaw), cos(yaw)*cos(roll)+sin(yaw)*sin(pitch), cos(pitch)*sin(roll);
    sin(yaw)*sin(roll)+cos(yaw)*cos(roll)*sin(pitch), cos(roll)*sin(yaw)*sin(pitch)-cos(yaw)*sin(roll), cos(roll)*cos(pitch)];

acc_RS = R_Global2RTBBody*vector;

== matlab function sim_quadrotor/DroneRS_Compensator/Estimator/EstimatorAttitude ==
  data: sensorIMU_datin input; yawVIS_datin input; validVIS_flagin input; gvecInit_datin input; att_estimout output; dt input; datt_estimout output; w_euler output
function [att_estimout,datt_estimout,w_euler] = fcn(sensorIMU_datin,yawVIS_datin,validVIS_flagin, gvecInit_datin,dt)
persistent yaw_cur pitch_cur roll_cur

p = sensorIMU_datin(4);
q = sensorIMU_datin(5);
r = sensorIMU_datin(6);

g = norm(gvecInit_datin,2);

if isempty(yaw_cur)
   yaw_cur = 0;
end
if isempty(pitch_cur)
   pitch_cur = 0;
end
if isempty(roll_cur)
   roll_cur = 0;
end


accvsGyro     = 0.001;
[yaw,pitch,roll,w_euler,forceMagnitudeApprox]= complimentaryfilter(yaw_cur, pitch_cur, roll_cur, g,dt,sensorIMU_datin, yawVIS_datin,validVIS_flagin,accvsGyro);
yaw_cur = yaw;
pitch_cur = pitch;
roll_cur = roll;

att_estimout = [yaw,pitch,roll]';
datt_estimout = [p,q,r]';

== matlab function sim_quadrotor/DroneRS_Compensator/Estimator/EstimatorXYPosition/EstimatorXYPosition/OutlierHandling/abs ==
  data: vec input; y output
function y = fcn(vec)
y = norm(vec,2);
